simulink model "HGO_robot_CASE_II"  (R2024a)
settings: Solver=FixedStepAuto  StartTime=0.0  StopTime=TF  FixedStep=Ts  MaxStep=1e-2  RelTol=1e-3
InitFcn:
  | HGO_parameters_Case_II
StopFcn:
  | results
values from neighbouring files (symbols this model uses):
  Gamma = eval([sol.G_11 sol.G_12 sol.G_13 sol.G_14 ... (first row only)    [HGO_parameters_Case_I.m]    (also in HGO_parameters_Case_II.m; HGO_parameters_Case_III.m)
  Kd = place(Ad,Bd,[0.9 0.95 0.95 0.9])    [HGO_parameters_Case_I.m]    (also in HGO_parameters_Case_II.m = place(Ad,Bd,[0.62 0.6 0.62 0.6]); HGO_parameters_Case_III.m = place(Ad,Bd,[0.92 0.95 0.95 0.92]))
  Pi = eval([sol.P_11 sol.P_12 sol.P_13 sol.P_14 ... (first row only)    [HGO_parameters_Case_I.m]    (also in HGO_parameters_Case_II.m; HGO_parameters_Case_III.m)
  Q = blkdiag(Q1,Q2)    [HGO_parameters_Case_I.m]    (also in HGO_parameters_Case_II.m; HGO_parameters_Case_III.m)
  SHd = blkdiag(H1d,H2d)    [HGO_parameters_Case_I.m]    (also in HGO_parameters_Case_II.m; HGO_parameters_Case_III.m)
  Sid = blkdiag(S1d,S2d)    [HGO_parameters_Case_I.m]    (also in HGO_parameters_Case_II.m; HGO_parameters_Case_III.m)
  t1 = (t1_op)    [HGO_parameters_Case_I.m]    (also in HGO_parameters_Case_II.m; HGO_parameters_Case_III.m = 1.9948)
  t1_ini = 1.4941    [HGO_parameters_Case_I.m]    (also in HGO_parameters_Case_II.m; HGO_parameters_Case_III.m = theta_1b(1))
  t2 = (t2_op)    [HGO_parameters_Case_I.m]    (also in HGO_parameters_Case_II.m; HGO_parameters_Case_III.m = -2.41)
  t2_ini = -1.9134    [HGO_parameters_Case_I.m]    (also in HGO_parameters_Case_II.m; HGO_parameters_Case_III.m = theta_2b(2))
  Ts = 0.001    [HGO_parameters_Case_I.m]    (also in HGO_parameters_Case_II.m = 0.0005; HGO_parameters_Case_III.m = TF/length(tiempo))
  ue = [u1;u2]    [HGO_parameters_Case_I.m]    (also in HGO_parameters_Case_II.m; HGO_parameters_Case_III.m)
  X = l1 * cos(THETA1) + l2 * cos(THETA1 + THETA2)    [HGO_parameters_Case_I.m]    (also in HGO_parameters_Case_II.m; HGO_parameters_Case_III.m)
  Y = l1 * sin(THETA1) + l2 * sin(THETA1 + THETA2)    [HGO_parameters_Case_I.m]    (also in HGO_parameters_Case_II.m; HGO_parameters_Case_III.m)
undefined symbols (not defined in the file or in its folder): Z
libraries: sm_lib x11, nesl_utility x9
Description:
  | Generación de una señal por un exosistema con la forma de un observador de alta ganacia que se produce de identificar una señal medida, en este caso el valor en el tiempo para que el robot genere una línea
settings Model: Creator=jesus  LastModifiedBy=ricar
settings SolverCC: AlgebraicLoopSolver=TrustRegion
settings OptimizationCC: ReuseModelBlockBuffer=off
settings DebuggingCC: UnconnectedInputMsg=warning  UnconnectedOutputMsg=warning  UnconnectedLineMsg=warning
settings ModelReferenceCC: EnableRefExpFcnMdlSchedulingChecks=on
settings RTWCC: GPUComputeCapability=3.5
settings ExplorerConfigSet: InternalSimMechanicsExplorerSettings="<ExplorerConfiguration><canonicalview>planar_xy</canonicalview><AnimationSetting><BasePlaybackSpeed>1.0</BasePlaybackSpeed><PlaybackSpeedFactor>1.0</PlaybackSpeedFactor></AnimationSetting><TilePanel><TileInfo><Tiles Columns=\"1\" Count=\"1\" Rows=\"1\"><Column Weight=\"1\"/><Row Weight=\"1\"/><Tile Height=\"1\" Width=\"1\" X=\"0\" Y=\"0\"/></Tiles></TileInfo><SceneInfo><SceneViewer><BGColor><R>0.60000002384185791</R><G>0.60000002384185791</G><B>0.60000002384185791</B></BGColor><Camera><DoPerspective>off</DoPerspective><Position><X>0.0505182147026062012</X><Y>0.371693924069404547</Y><Z>1.00000000000000044</Z></Position><Center><X>0.0505182147026062012</X><Y>0.371693924069404547</Y><Z>4.44089209850062616e-16</Z></Center><Up><X>0</X><Y>1</Y><Z>0</Z></Up><ViewLimDist>1</ViewLimDist><YLim>0.389655273556709314</YLim><XLim>0.468666828160062887</XLim></Camera></SceneViewer></SceneInfo></TilePanel><MechEditorPanel><Cameras/><GfxPanelCameraMap/><VideoCreator><PlaybackSpeedRatio>1.0</PlaybackSpeedRatio><FrameRate>30</FrameRate><VideoFormat>Motion JPEG AVI</VideoFormat><FrameSize>auto</FrameSize></VideoCreator></MechEditorPanel></ExplorerConfiguration>"

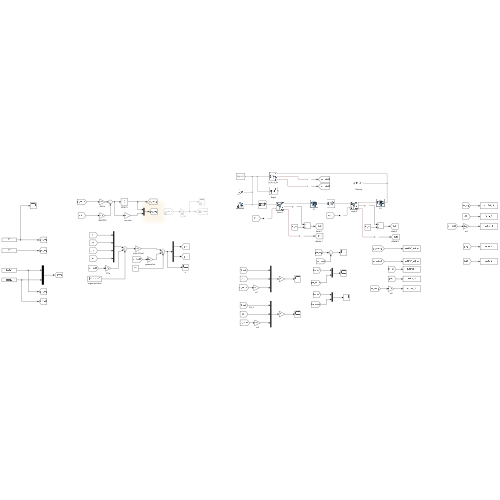
[thumbnail: Simulink's stored preview of the top-level diagram]
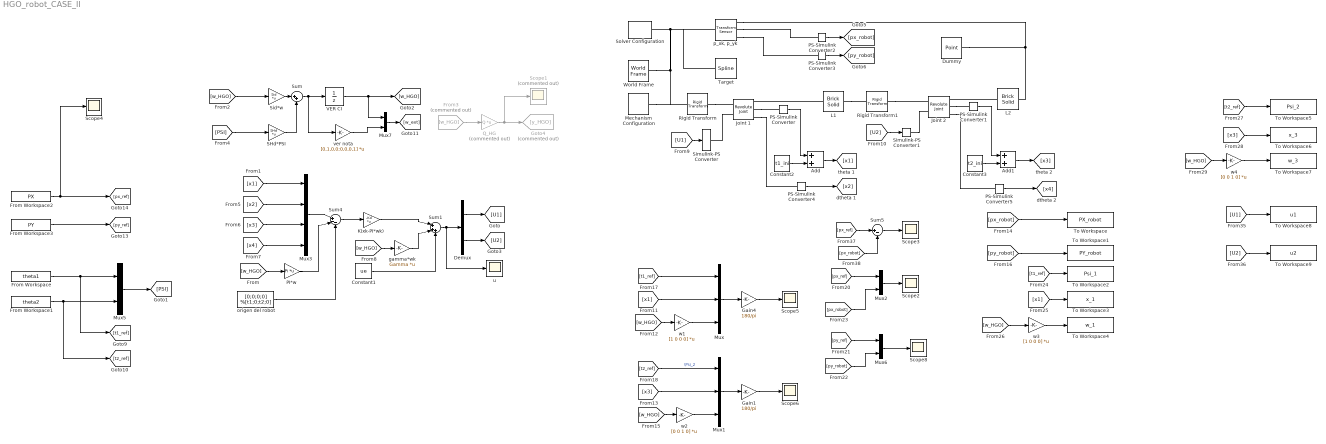
== system HGO_robot_CASE_II ==
  Add : Sum
  Add1 : Sum
  Constant1 : Constant  Value=ue
  Constant2 : Constant  Value=t1_ini
  Constant3 : Constant  Value=t2_ini
  Demux : Demux  Outputs=2
  Dummy : sm_lib/Curves and Surfaces/Point  GraphicType=Marker  MarkerShape=Sphere  MarkerSize=20  GraphicVisPropType=SimpleVisualProperties  GraphicDiffuseColor=[0.5 0.5 0.5]  GraphicOpacity=1.0  GraphicSpecularColor=[0.5 0.5 0.5 1.0]  GraphicAmbientColor=[0.15 0.15 0.15 1.0]  GraphicEmissiveColor=[0.0 0.0 0.0 1.0]  GraphicShininess=75
  From Workspace : FromWorkspace  VariableName=theta1  SampleTime=Ts
  From Workspace1 : FromWorkspace  VariableName=theta2  SampleTime=Ts
  From Workspace2 : FromWorkspace  VariableName=PX  SampleTime=Ts
  From Workspace3 : FromWorkspace  VariableName=PY  SampleTime=Ts
  From3 : From  Commented=on  GotoTag=w_HGO
  Gain1 : Gain  Gain=180/pi
  Gain4 : Gain  Gain=180/pi
  Goto4 : Goto  Commented=on  GotoTag=y_HGO
  Joint 1 : sm_lib/Joints/Revolute Joint  JointMode=Normal  CompositeWrenchDir=FollowerOnBase  CompositeWrenchFrame=BaseFrame  SenseConstraintForce=off  SenseConstraintTorque=off  SenseTotalForce=off  SenseTotalTorque=off  PositionTargetSpecify=off  PositionTargetPriority=High  PositionTargetValue=0  PositionTargetValueUnits=deg  VelocityTargetSpecify=off  VelocityTargetPriority=High  VelocityTargetValue=0  VelocityTargetValueUnits=deg/s  EquilibriumPosition=0  EquilibriumPositionUnits=deg  SpringStiffness=0  SpringStiffnessUnits=N*m/deg  DampingCoefficient=0  DampingCoefficientUnits=N*m/(deg/s)  LowerLimitSpecify=off  LowerLimitBound=-90  LowerLimitBoundUnits=deg  LowerLimitStiffness=1e4  LowerLimitStiffnessUnits=N*m/deg  LowerLimitDamping=10  LowerLimitDampingUnits=N*m/(deg/s)  LowerLimitTransitionRegionWidth=0.1  LowerLimitTransitionRegionWidthUnits=deg  UpperLimitSpecify=off  UpperLimitBound=90  UpperLimitBoundUnits=deg  UpperLimitStiffness=1e4  UpperLimitStiffnessUnits=N*m/deg  UpperLimitDamping=10  UpperLimitDampingUnits=N*m/(deg/s)  UpperLimitTransitionRegionWidth=0.1  UpperLimitTransitionRegionWidthUnits=deg  TorqueActuationMode=InputTorque  MotionActuationMode=ComputedMotion  SensePosition=on  SenseVelocity=on  SenseAcceleration=off  SenseTorqueForce=off  SenseLowerLimitTorqueForce=off  SenseUpperLimitTorqueForce=off
  Joint 2 : sm_lib/Joints/Revolute Joint  JointMode=Normal  CompositeWrenchDir=FollowerOnBase  CompositeWrenchFrame=BaseFrame  SenseConstraintForce=off  SenseConstraintTorque=off  SenseTotalForce=off  SenseTotalTorque=off  PositionTargetSpecify=off  PositionTargetPriority=High  PositionTargetValue=0  PositionTargetValueUnits=deg  VelocityTargetSpecify=off  VelocityTargetPriority=High  VelocityTargetValue=0  VelocityTargetValueUnits=deg/s  EquilibriumPosition=0  EquilibriumPositionUnits=deg  SpringStiffness=0  SpringStiffnessUnits=N*m/deg  DampingCoefficient=0  DampingCoefficientUnits=N*m/(deg/s)  LowerLimitSpecify=off  LowerLimitBound=-90  LowerLimitBoundUnits=deg  LowerLimitStiffness=1e4  LowerLimitStiffnessUnits=N*m/deg  LowerLimitDamping=10  LowerLimitDampingUnits=N*m/(deg/s)  LowerLimitTransitionRegionWidth=0.1  LowerLimitTransitionRegionWidthUnits=deg  UpperLimitSpecify=off  UpperLimitBound=90  UpperLimitBoundUnits=deg  UpperLimitStiffness=1e4  UpperLimitStiffnessUnits=N*m/deg  UpperLimitDamping=10  UpperLimitDampingUnits=N*m/(deg/s)  UpperLimitTransitionRegionWidth=0.1  UpperLimitTransitionRegionWidthUnits=deg  TorqueActuationMode=InputTorque  MotionActuationMode=ComputedMotion  SensePosition=on  SenseVelocity=on  SenseAcceleration=off  SenseTorqueForce=off  SenseLowerLimitTorqueForce=off  SenseUpperLimitTorqueForce=off
  K(xk-PI*wk) : Gain  Gain=-Kd  Multiplication=Matrix(K*u)
  L1 : sm_lib/Body Elements/Brick Solid  BrickDimensions=[0.5 .01 .01]  BrickDimensionsUnits=m  ExportEntireGeometry=off  InertiaType=CalculateFromGeometry  BasedOnType=Mass  Density=1000  DensityUnits=kg/m^3  Mass=.4  MassUnits=kg  CenterOfMass=[0 0 0]  CenterOfMassUnits=m  MomentsOfInertia=[1 1 1]  MomentsOfInertiaUnits=kg*m^2  ProductsOfInertia=[0 0 0]  ProductsOfInertiaUnits=kg*m^2  GraphicType=FromGeometry  MarkerShape=Sphere  MarkerSize=10  GraphicVisPropType=SimpleVisualProperties  GraphicDiffuseColor=[0.5 0.5 0.5]  GraphicOpacity=1.0  GraphicSpecularColor=[0.5 0.5 0.5 1.0]  GraphicAmbientColor=[0.15 0.15 0.15 1.0]  GraphicEmissiveColor=[0.0 0.0 0.0 1.0]  GraphicShininess=75  DoExposeReferenceFrame=off  SerializedFrames=<Frames><Frame><Id>Frame1</Id><Value><Name>F1</Name><Origin><Source>GeometricFeature</Source><FeatureName>-x surface</FeatureName></Origin><PrimaryAxis><DefinedDirection>+Z</DefinedDirection><Source>ReferenceFrame</Source><SourceDirection>+Z</SourceDirection><FeatureName></FeatureName></PrimaryAxis><SecondaryAxis><DefinedDirection>+X</DefinedDirection><Source>ReferenceFrame</Source><SourceDirection>+X</SourceDirection><FeatureName></FeatureName></SecondaryAxis></Value></Frame><Frame><Id>Frame2</Id><Value><Name>F2</Name><Origin><Source>GeometricFeature</Source><FeatureName>+x surface</FeatureName></Origin><PrimaryAxis><DefinedDirection>+Z</DefinedDirection><Source>ReferenceFrame</Source><SourceDirection>+Z</SourceDirection><FeatureName></FeatureName></PrimaryAxis><SecondaryAxis><DefinedDirection>+X</DefinedDirection><Source>ReferenceFrame</Source><SourceDirection>+X</SourceDirection><FeatureName></FeatureName></SecondaryAxis></Value></Frame></Frames>
  L2 : sm_lib/Body Elements/Brick Solid  BrickDimensions=[0.5 .01 .01]  BrickDimensionsUnits=m  ExportEntireGeometry=off  InertiaType=CalculateFromGeometry  BasedOnType=Mass  Density=1000  DensityUnits=kg/m^3  Mass=.3  MassUnits=kg  CenterOfMass=[0 0 0]  CenterOfMassUnits=m  MomentsOfInertia=[1 1 1]  MomentsOfInertiaUnits=kg*m^2  ProductsOfInertia=[0 0 0]  ProductsOfInertiaUnits=kg*m^2  GraphicType=FromGeometry  MarkerShape=Sphere  MarkerSize=10  GraphicVisPropType=SimpleVisualProperties  GraphicDiffuseColor=[0.5 0.5 0.5]  GraphicOpacity=1.0  GraphicSpecularColor=[0.5 0.5 0.5 1.0]  GraphicAmbientColor=[0.15 0.15 0.15 1.0]  GraphicEmissiveColor=[0.0 0.0 0.0 1.0]  GraphicShininess=75  DoExposeReferenceFrame=off  SerializedFrames=<Frames><Frame><Id>Frame1</Id><Value><Name>F1</Name><Origin><Source>GeometricFeature</Source><FeatureName>-x surface</FeatureName></Origin><PrimaryAxis><DefinedDirection>+Z</DefinedDirection><Source>ReferenceFrame</Source><SourceDirection>+Z</SourceDirection><FeatureName></FeatureName></PrimaryAxis><SecondaryAxis><DefinedDirection>+X</DefinedDirection><Source>ReferenceFrame</Source><SourceDirection>+X</SourceDirection><FeatureName></FeatureName></SecondaryAxis></Value></Frame><Frame><Id>Frame2</Id><Value><Name>F2</Name><Origin><Source>GeometricFeature</Source><FeatureName>+x surface</FeatureName></Origin><PrimaryAxis><DefinedDirection>+Z</DefinedDirection><Source>ReferenceFrame</Source><SourceDirection>+Z</SourceDirection><FeatureName></FeatureName></PrimaryAxis><SecondaryAxis><DefinedDirection>+X</DefinedDirection><Source>ReferenceFrame</Source><SourceDirection>+X</SourceDirection><FeatureName></FeatureName></SecondaryAxis></Value></Frame></Frames>
  Mechanism Configuration : sm_lib/Utilities/Mechanism Configuration  UniformGravity=Constant  GravityVector=[0 -9.80665 0]  GravityVectorUnits=m/s^2  LinearizationDelta=0.001  JointModeTransitionNonlinearIterations=2
  Mux : Mux  Inputs=3
  Mux1 : Mux  Inputs=3
  Mux{2,5..7} (4 alike) : Mux  Inputs=2
  Mux3 : Mux
  PI*w : Gain  Gain=Pi  Multiplication=Matrix(K*u)
  PS-Simulink Converter : nesl_utility/PS-Simulink Converter  PhysicalDomain=network_engine_domain  SubClassName=ps_output  LeftPortType=input  RightPortType=output  PseudoPeriodic=off  Frequencies=[]  VectorFormat=1-D array  Unit=inherit  AffineConversion=off
  PS-Simulink Converter1 : nesl_utility/PS-Simulink Converter  PhysicalDomain=network_engine_domain  SubClassName=ps_output  LeftPortType=input  RightPortType=output  PseudoPeriodic=off  Frequencies=[]  VectorFormat=1-D array  Unit=inherit  AffineConversion=off
  PS-Simulink Converter{2..5} (4 alike) : nesl_utility/PS-Simulink Converter  PhysicalDomain=network_engine_domain  SubClassName=ps_output  LeftPortType=input  RightPortType=output  PseudoPeriodic=off  Frequencies=[]  VectorFormat=inherit  Unit=inherit  AffineConversion=off
  "Q_HG " : Gain  Commented=on  Gain=Q  Multiplication=Matrix(K*u)
  Rigid Transform : sm_lib/Frames and Transforms/Rigid Transform  RotationMethod=StandardAxis  FollAlignAxisA=+X  BaseAlignAxisA=+Y  FollAlignAxisB=+Y  BaseAlignAxisB=+Z  RotationStandardAxis=+Z  RotationAngle=t1_ini  RotationAngleUnits=rad  RotationArbitraryAxis=[0 0 1]  RotationSequenceAxes=FollowerAxes  RotationSequence=XYX  RotationSequenceAngles=[0 0 0]  RotationSequenceAnglesUnits=deg  RotationMatrix=[1 0 0; 0 1 0; 0 0 1]  Quaternion=[1 0 0 0]  TranslationMethod=None  TranslationCartesianOffset=[0 0 0]  TranslationCartesianOffsetUnits=m  TranslationStandardAxis=+Z  TranslationStandardOffset=0  TranslationStandardOffsetUnits=m  TranslationROffset=0  TranslationROffsetUnits=m  TranslationThetaOffset=0  TranslationThetaOffsetUnits=deg  TranslationZOffset=0  TranslationZOffsetUnits=m
  Rigid Transform1 : sm_lib/Frames and Transforms/Rigid Transform  RotationMethod=StandardAxis  FollAlignAxisA=+X  BaseAlignAxisA=+Y  FollAlignAxisB=+Y  BaseAlignAxisB=+Z  RotationStandardAxis=+Z  RotationAngle=t2_ini  RotationAngleUnits=rad  RotationArbitraryAxis=[0 0 1]  RotationSequenceAxes=FollowerAxes  RotationSequence=XYX  RotationSequenceAngles=[0 0 0]  RotationSequenceAnglesUnits=deg  RotationMatrix=[1 0 0; 0 1 0; 0 0 1]  Quaternion=[1 0 0 0]  TranslationMethod=None  TranslationCartesianOffset=[0 0 0]  TranslationCartesianOffsetUnits=m  TranslationStandardAxis=+Z  TranslationStandardOffset=0  TranslationStandardOffsetUnits=m  TranslationROffset=0  TranslationROffsetUnits=m  TranslationThetaOffset=0  TranslationThetaOffsetUnits=deg  TranslationZOffset=0  TranslationZOffsetUnits=m
  "SHd*PSI " : Gain  Gain=SHd  Multiplication=Matrix(K*u)
  Scope1 : Scope  Commented=on
  Scope{2..6,8} (6 alike) : Scope
  Sid*w : Gain  Gain=Sid  Multiplication=Matrix(K*u)
  Simulink-PS Converter : nesl_utility/Simulink-PS Converter  PhysicalDomain=network_engine_domain  SubClassName=ps_input  LeftPortType=input  RightPortType=output  PseudoPeriodic=off  Frequencies=[]  NoiseDistribution=none  NoiseParameters=[]  Unit=1  AffineConversion=on  FilteringAndDerivatives=provide  SimscapeFilterOrder=1  InputFilterTimeConstant=Ts  UdotUserProvided=0
  Simulink-PS Converter1 : nesl_utility/Simulink-PS Converter  PhysicalDomain=network_engine_domain  SubClassName=ps_input  LeftPortType=input  RightPortType=output  PseudoPeriodic=off  Frequencies=[]  NoiseDistribution=none  NoiseParameters=[]  Unit=1  AffineConversion=on  FilteringAndDerivatives=provide  SimscapeFilterOrder=1  InputFilterTimeConstant=Ts  UdotUserProvided=0
  Solver Configuration : nesl_utility/Solver Configuration  PhysicalDomain=network_engine_domain  SubClassName=solver  LeftPortType=input  RightPortType=generic  Tones=[]  Harmonics=[]  SimulateNoise=off  Profile=off  UseLocalSampling=off  EnableSwitchedLinearOptims=on  FrequencyDomain=off  UseCCode=off  RelTol=0.001  AbsTol=0.001  MinStep=1e-09  ToWorkspace=off  RevertToSquareIcSolve=off  NumHomotopyIterations=100  PhasorMode=off  PhasorModeNumHarmonics=1  ConsistencySolver=NEWTON_XTOL_AFTER_FTOL  IndexReductionMethod=DerivativeReplacement  DoDC=off  ResidualTolerance=1e-09  ConsistencyTolSource=GLOBAL  ConsistencyAbsTol=0.001  ConsistencyRelTol=0.001  ConsistencyTolFactor=0.001  UseLocalSolver=off  LocalSolverChoice=NE_BACKWARD_EULER_ADVANCER  ResolveIndetEquations=on  FunctionEvalNumThread=1  LocalSolverSampleTime=0.001  DoFixedCost=off  MaxNonlinIter=3  MaxModeIter=2  ComputeImpulses=off  ImpulseIterations=2  LinearAlgebra=auto  LinearAlgebraNumThread=0  EquationFormulation=NE_TIME_EF  DelaysMemoryBudget=1024  AutomaticFiltering=on  FilteringTimeConstant=0.001  PartitionStorageMethod=AS_NEEDED  PartitionMemoryBudget=1024  PartitionMethod=ROBUST  MultibodyUseLocalSolver=off  MultibodyLocalSolverChoice=ODE1  MultibodyLocalSolverSampleTime=0.001
  Sum : Sum  Inputs=|++
  Sum1 : Sum  Inputs=|+++
  Sum4 : Sum  Inputs=|+--
  Sum5 : Sum  Inputs=|+-
  Target : sm_lib/Curves and Surfaces/Spline  DataPoints=traj_adj  DataPointsUnits=m  EndConditionType=Natural  GraphicType=FromGeometry  MarkerShape=Frame  MarkerSize=10  GraphicVisPropType=AdvancedVisualProperties  GraphicDiffuseColor=[0.0 0.0 0.0]  GraphicOpacity=1.0  GraphicSpecularColor=[0.5 0.5 0.5 1.0]  GraphicAmbientColor=[0.15 0.15 0.15 1.0]  GraphicEmissiveColor=[0.0 0.0 0.0 1.0]  GraphicShininess=75
  To Workspace : ToWorkspace  VariableName=PX_robot  SampleTime=-1
      settings: Save2DSignal=2-D array (concatenate along first dimension)
  To Workspace1 : ToWorkspace  VariableName=PY_robot  SampleTime=-1
      settings: Save2DSignal=2-D array (concatenate along first dimension)
  To Workspace2 : ToWorkspace  VariableName=Psi_1  SampleTime=-1
  To Workspace3 : ToWorkspace  VariableName=x_1  SampleTime=-1
  To Workspace4 : ToWorkspace  VariableName=w_1  SampleTime=-1
  To Workspace5 : ToWorkspace  VariableName=Psi_2  SampleTime=-1
  To Workspace6 : ToWorkspace  VariableName=x_3  SampleTime=-1
  To Workspace7 : ToWorkspace  VariableName=w_3  SampleTime=-1
  To Workspace8 : ToWorkspace  VariableName=u1  SampleTime=-1
  To Workspace9 : ToWorkspace  VariableName=u2  SampleTime=-1
  VER CI : UnitDelay  InitialCondition=[t1_ini;0;t2_ini;0]%zeros(4,1)  SampleTime=Ts  HasFrameUpgradeWarning=on
  World Frame : sm_lib/Frames and Transforms/World Frame
  gamma*wk : Gain  Gain=Gamma  Multiplication=Matrix(K*u)
  origen del robot : Constant  Value=[0;0;0;0] %[t1;0;t2;0]
  "p_xk, p_yk" : sm_lib/Frames and Transforms/Transform Sensor  MeasurementFrame=World  RotationSequence=XYX  SenseAngle=off  SenseAxis=off  SenseQ=off  SenseR=off  SenseRotationSequence=off  SenseOmegaX=off  SenseOmegaY=off  SenseOmegaZ=off  SenseOmega=off  SenseQDot=off  SenseRDot=off  SenseRotationSequenceDot=off  SenseAlphaX=off  SenseAlphaY=off  SenseAlphaZ=off  SenseAlpha=off  SenseQDDot=off  SenseRDDot=off  SenseX=on  SenseY=on  SenseZ=off  SenseXYZ=off  SenseRad=off  SenseAzim=off  SenseDist=off  SenseInc=off  SenseXDot=off  SenseYDot=off  SenseZDot=off  SenseXYZDot=off  SenseRadDot=off  SenseAzimDot=off  SenseDistDot=off  SenseIncDot=off  SenseXDDot=off  SenseYDDot=off  SenseZDDot=off  SenseXYZDDot=off  SenseRadDDot=off  SenseAzimDDot=off  SenseDistDDot=off  SenseIncDDot=off
  u : Scope
  ver nota : Gain  Description=|  Gain=[0,1,0,0;0,0,0,1]  Multiplication=Matrix(K*u)
      | esto se agregó para cuando se usa el contro no lineal, 
      | para obtener las aceleraciones de las articulaciones, generamos el omega extendido
  w1 : Gain  Gain=[1 0 0 0]  Multiplication=Matrix(K*u)
  w2 : Gain  Gain=[0 0 1 0]  Multiplication=Matrix(K*u)
  w3 : Gain  Gain=[1 0 0 0]  Multiplication=Matrix(K*u)
  w4 : Gain  Gain=[0 0 1 0]  Multiplication=Matrix(K*u)
  wires:
  [w_HGO] -> Sid*w/1
  Sid*w/1 -> Sum/1
  VER CI/1 -> Mux7/1, [w_HGO]
  From3/1 -> "Q_HG "/1
  "Q_HG "/1 -> Scope1/1, Goto4/1
  Mux/1 -> Gain4/1
  Gain4/1 -> Scope5/1
  Gain1/1 -> Scope6/1
  Mux1/1 -> Gain1/1
  PI*w/1 -> Sum4/2
  Mux5/1 -> [PSI]
  "SHd*PSI "/1 -> Sum/2
  [PSI] -> "SHd*PSI "/1
  [w_HGO] -> PI*w/1
  PS-Simulink Converter4/1 -> [x2]
  PS-Simulink Converter5/1 -> [x4]
  Sum4/1 -> K(xk-PI*wk)/1
  K(xk-PI*wk)/1 -> Sum1/1
  [w_HGO] -> gamma*wk/1
  Demux/1 -> [U1]
  Demux/2 -> [U2]
  Add/1 -> [x1]
  PS-Simulink Converter/1 -> Add/1
  Constant2/1 -> Add/2
  [U1] -> Simulink-PS Converter/1
  [U2] -> Simulink-PS Converter1/1
  Constant1/1 -> Sum1/3
  Mux3/1 -> Sum4/1
  Sum1/1 -> u/1, Demux/1
  From Workspace/1 -> [t1_ref], Mux5/1
  From Workspace1/1 -> Mux5/2, [t2_ref]
  PS-Simulink Converter1/1 -> Add1/1
  Add1/1 -> [x3]
  Constant3/1 -> Add1/2
  [x1] -> Mux3/1
  [x2] -> Mux3/2
  [x3] -> Mux3/3
  [x4] -> Mux3/4
  Mux2/1 -> Scope2/1
  Mux6/1 -> Scope8/1
  Sum/1 -> ver nota/1, VER CI/1
  ver nota/1 -> Mux7/2
  Mux7/1 -> [w_ext]
  [w_HGO] -> w1/1
  [w_HGO] -> w2/1
  PS-Simulink Converter2/1 -> [px_robot]
  PS-Simulink Converter3/1 -> [py_robot]
  [py_ref] -> Mux6/1
  [px_ref] -> Mux2/1
  [px_robot] -> Mux2/2
  [py_robot] -> Mux6/2
  [px_robot] -> To Workspace/1
  [py_robot] -> To Workspace1/1
  [t1_ref] -> Mux/1
  [t2_ref] -> Mux1/1  "\\Psi_2"
  w2/1 -> Mux1/3
  [x3] -> Mux1/2
  w1/1 -> Mux/3
  [x1] -> Mux/2
  [x1] -> To Workspace3/1
  [t1_ref] -> To Workspace2/1
  [t2_ref] -> To Workspace5/1
  [x3] -> To Workspace6/1
  [w_HGO] -> w4/1
  w3/1 -> To Workspace4/1
  [w_HGO] -> w3/1
  w4/1 -> To Workspace7/1
  gamma*wk/1 -> Sum1/2
  origen del robot/1 -> Sum4/3
  [U1] -> To Workspace8/1
  [U2] -> To Workspace9/1
  Sum5/1 -> Scope3/1
  [px_robot] -> Sum5/2
  [px_ref] -> Sum5/1
  From Workspace2/1 -> [px_ref], Scope4/1
  From Workspace3/1 -> [py_ref]
  connections:
  L1/LConn1 -- Joint 1/RConn1
  Joint 1/RConn2 -- PS-Simulink Converter/LConn1
  World Frame/RConn1 -- Target/LConn1 -- "p_xk, p_yk"/LConn1 -- Solver Configuration/RConn1 -- Rigid Transform/LConn1 -- Mechanism Configuration/RConn1
  Joint 2/RConn2 -- PS-Simulink Converter1/LConn1
  L2/LConn1 -- Joint 2/RConn1
  L1/RConn1 -- Rigid Transform1/LConn1
  "p_xk, p_yk"/RConn1 -- Dummy/LConn1 -- L2/RConn1
  Joint 1/RConn3 -- PS-Simulink Converter4/LConn1
  Joint 2/RConn3 -- PS-Simulink Converter5/LConn1
  Joint 1/LConn2 -- Simulink-PS Converter/RConn1
  Simulink-PS Converter1/RConn1 -- Joint 2/LConn2
  Rigid Transform/RConn1 -- Joint 1/LConn1
  "p_xk, p_yk"/RConn2 -- PS-Simulink Converter2/LConn1
  "p_xk, p_yk"/RConn3 -- PS-Simulink Converter3/LConn1
  Rigid Transform1/RConn1 -- Joint 2/LConn1
